simulink model "Lombardini_dual_fuel"  (R2024b)
settings: Solver=FixedStepAuto  StartTime=0.0  StopTime=2000  RelTol=1e-3  EnableMultiTasking=on
PreLoadFcn:
  | try, eval([bdroot '_setup']); catch, eval('model_setup', ''); end
InitFcn:
  | try, eval([bdroot '_setup']); catch, eval('model_setup', ''); end
model workspace (MAT data in the model file):
  PID_rpm = [1000 2000 3000 4000]
undefined symbols (not defined in the file): ECU555, motohawk_build_version, motohawk_get_target_image, motohawk_target_type, motohawk_trunc_name, motohawk_vardec_path
libraries: MotoHawk_lib x118, motohawk_annotations_lib x23, dspstat3 x13, motohawk_examples_lib x1, MotoHawk_Protocols_lib x1
(part 1 of 5)
CloseFcn:
  | try, eval([bdroot '_close']); catch, eval('model_close', ''); end
Description:
  | Lombardini_dual_fuel
settings Model: MotoHawkBuildVersion=000  MotoHawkBuildStats=struct('TotalFLASH',{0},'TotalEEPROM',{0},'TotalRAM',{0},'AppFLASH',{0},'AppEEPROM',{0},'AppRAM',{0},'HeapRAM',{0},'BuildSuccessCount',{0},'BuildErrorCount',{0})  MotoHawkModelSavedName=Lombardini_dual_fuel  MotoHawkModelGUID=DD803FFC-3B74-4B09-85B7-E854500213FD  MotoHawkModelOpenTime=2025 8 5 14 36 14.209  MotoHawkModelElapsedTime=1228077.779  MotoHawkBuildInfo=struct('model_name',{'motohawk_template_model'},'motohawk_version',{'0.8.4_beta1'},'motohawk_component_version',{'0.0.3'},'matlab_version',{'6.5.1'},'build_version',{'000'},'layout_type',{'DEV'},'eri_table0_rev',{9},'max_eri_table_size',{255},'fptype',{0},'fgnd_base_period_ms',{5},'bgnd_base_period_ms',{50},'module_type',{'ECU555-80'},'processor_family',{'PPC'},'processor_type',{'MPC555'},'toolchain',{'GHS3.6'},'component',{0},'resource_file',{'PCM555Resources.h'},'archive_file',{'PCM.a'},'enable_build',{1},'flash_size',{458752},'ee_size',{8192},'ram_size',{26624},'decram_size',{0},'module_memory_def',{'MPC555_ModMemoryDef_Dev'},'use_debug_vardecs',{1},'root_build_dir',{'C:\MotoTron\MOTOHA~3\Blocks\Project'},'build_dir',{'C:\MotoTron\MOTOHA~3\Blocks\Project\motohawk_template_model_Build'},'dll_name',{'motohawk__000'},'srz_name',{'motohawk_template_model_000'},'fgnd_stack_size',{3072},'fgnd_angle_stack_size',{0},'bgnd_stack_size',{2048},'idle_stack_size',{1024},'irq_stack_size',{1536},'heap_size',{4096},'install_dll_dir',{'C:\ECUFiles\TDBDLL\'},'install_srz_dir',{'C:\ECUFiles\Programs\'},'motodevelopment_dir',{'C:\PROGRA~1\MotoTron\DEVELO~1\'},'motohawk_dir',{'C:\MotoTron\MOTOHA~3'},'ghs_dir',{'C:\GHS\ppc36'},'cw_dir',{'C:\Program Files\Freescale\CW for HC12 V4.5'},'matlab_root',{'C:\MATLAB6p5p1'},'model_guid',{'a528c725-4135-4734-9f-2c-07-29-37-5b-38'},'build_guid',{[]},'token_guid',{'6198A7A8FF044D4685C525ADFA06DAD5'})  MotoHawkBuildDirectory=C:\Users\ASUS\MATLAB\Projects\Lombardini_Hybrid\models\Lombardini_dual_fuel_Build  MotoHawkTargetDefnBlock=Lombardini_dual_fuel/motohawk_target_def1  MotoHawkCANInfo=struct('DefnArr',{struct('res_name',{'CAN_1'},'text_resource',{'(None)'},'IsSupportedMethodArr',{logical([0;0;0;0;0;0;0;0;0;0;0;0;0;0;0;0;0])})})  Creator=cspenc  LastModifiedBy=ASUS
settings ConfigSet: Description="This Simulink Configuration Set is preconfigured  for the MotoHawk target \"ECU555-48-0403\"."
settings SolverCC: AlgebraicLoopSolver=TrustRegion  AutoInsertRateTranBlk=on
settings DataIOCC: LimitDataPoints=on  SaveFormat=Array  ReturnWorkspaceOutputs=off
settings OptimizationCC: DefaultParameterBehavior=Inlined  InlineInvariantSignals=on  EnhancedBackFolding=on  InitFltsAndDblsToZero=on  NoFixptDivByZeroProtection=on  EfficientFloat2IntCast=on  LifeSpan=1  EfficientTunableParamExpr=on
settings DebuggingCC: AlgebraicLoopMsg=none  MergeDetectMultiDrivingBlocksExec=none  InheritedTsInSrcMsg=none  TasksWithSamePriorityMsg=none  ParamSuppressDoubleToSinglePrecisionLossMsg=on  ParamPrecisionLossAbsoluteDiffThreshold=0.5  UnconnectedInputMsg=warning  UnconnectedOutputMsg=warning  UnconnectedLineMsg=warning  ModelReferenceIOMismatchMessage=warning  SFUnexpectedBacktrackingDiag=warning  SFNoUnconditionalDefaultTransitionDiag=warning  SFExecutionAtInitializationDiag=none  UnitsInconsistencyMsg=none  ArithmeticOperatorsInVariantConditions=warning
settings HardwareCC: ProdBitPerPointer=32  ProdBitPerSizeT=32  ProdBitPerPtrDiffT=32  ProdLargestAtomicInteger=Integer  ProdIntDivRoundTo=Undefined  ProdEndianess=BigEndian  ProdWordSize=32  ProdHWDeviceType=Specified
settings ModelReferenceCC: UpdateModelReferenceTargets=IfOutOfDate  EnableRefExpFcnMdlSchedulingChecks=on  CheckModelReferenceTargetMessage=warning  ModelReferenceNumInstancesAllowed=Single  PropagateSignalLabelsOutOfModel=off
settings SFSimCC: SimCustomHeaderCode="#include \"FuelControl.h\""  SimUserSources=Code/Fuelcontrol.c  SimUserIncludeDirs=Code  SimUseLocalCustomCode=off  MATLABDynamicMemAlloc=off  CustomCodeUndefinedFunction=UseInterfaceOnly
settings RTWCC: Description=MotoHawk(tm) Rapid Prototyping  SystemTargetFile=motohawk_ert_rtw.tlc  MakeCommand=make_rtw_motohawk  TemplateMakefile=motohawk_ert_rtw.tmf  RTWUseLocalCustomCode=off  GPUComputeCapability=3.5
settings CodeAppCC: IgnoreCustomStorageClasses=off  MaxIdLength=100  CustomSymbolStrType=$N$R$M  CustomSymbolStrField=$H$N$M  StateflowObjectComments=on  InternalIdentifier=Classic
settings STFCustomTargetCC: MultiwordTypeDef=User defined  MultiwordLength=0  IncludeMdlTerminateFcn=off  CombineOutputUpdateFcns=on  SuppressErrorStatus=on  ERTCustomFileBanners=on  SupportContinuousTime=off  SupportNonInlinedSFcns=off  RemoveResetFunc=on  MATLABClassNameForMDSCustomization=Simulink.SoftwareTarget.ERTCustomization  SystemTargetFile=motohawk_ert_rtw.tlc
settings ERTTargetCC: MultiwordTypeDef=User defined  MultiwordLength=0  ParMdlRefBuildCompliant=off  CompOptLevelCompliant=off  ConcurrentExecutionCompliant=off  IncludeMdlTerminateFcn=off  SuppressErrorStatus=on  ModelStepFunctionPrototypeControlCompliant=off  CPPClassGenCompliant=off  UseToolchainInfoCompliant=off  ERTCustomFileTemplate=motohawk_file_process.tlc  ConvertIfToSwitch=off  SuppressUnreachableDefaultCases=off  DynamicArrayContainerType=coder::array
settings ConfigComp: CovMetricSettings=dw  CovSaveCumulativeToWorkspaceVar=on  CovSaveSingleToWorkspaceVar=on  CovExternalEMLEnable=off  CovSFcnEnable=off

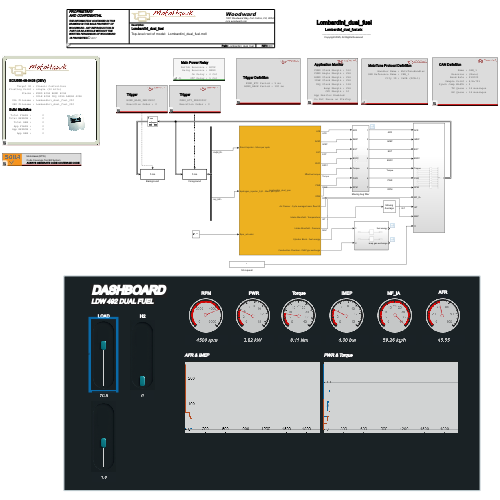
[thumbnail: Simulink's stored preview of the top-level diagram]
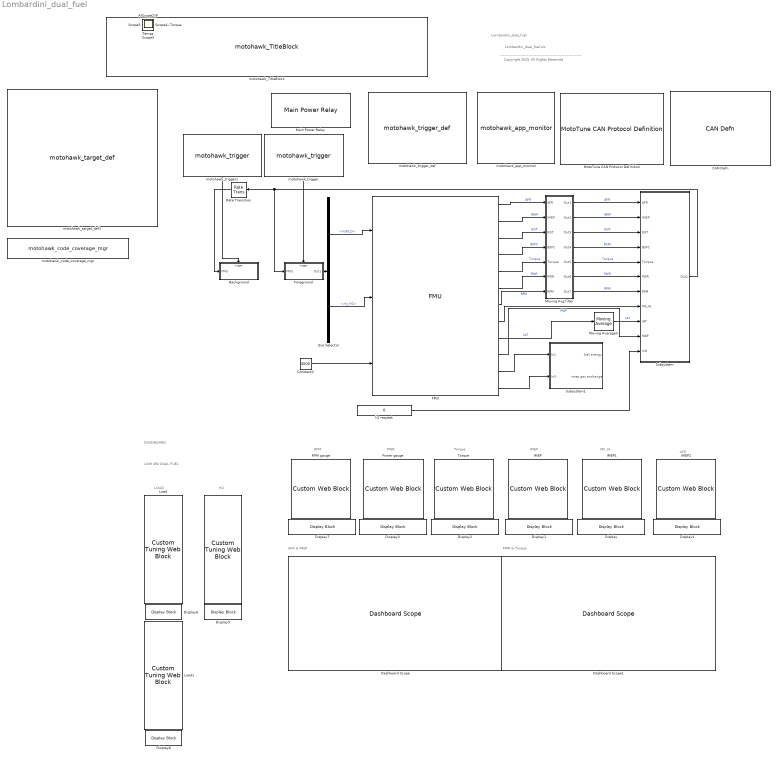
== system Lombardini_dual_fuel ==
  note: RPM
  note: Lombardini_dual_fuel
  note: Lombardini_dual_fuel.slx
  note: -------------------------------------------------------------
  note: Copyright 2025, All Rights Reserved
  note: PWR
  note: Torque
  note: IMEP
  note: MF_IA
  note: AFR
  note: LOAD
  note: H2
  note: DASHBOARD
  note: AFR & IMEP
  note: PWR & Torque
  note: LDW 492 DUAL FUEL
  . : CustomTuningWebBlock  LabelPosition=Hide  ShowInitialText=on  Configuration="{\"components\":[{\"name\":\"LinearScaleComponent\",\"settings\":{\"bounds\":{\"max\":1,\"min\":0,\"tickInterval\":\"auto\"},\"internalTickHeightScaleFactor\":0.66,\"labelColor\":[255,255,255],\"labelFont\":{\"font\":\"Arial\",\"fontSize\":12},\"labelOffset\":0.054,\"labelTransparency\":1,\"needleImage\":{\"size\":[216,346],\"src\":\"data:image\\/jpeg;base64,\\/9j\\/60nfSlCyAAAAAAEAAEnVanVtYgAAAB5qdW1kYzJwYQARABCAAACqADibcQNjMnBhAAAANxNqdW1iAAAAR2p1bWRjMm1hABEAEIAAAKoAOJtxA3VybjpjMnBhOmZjZjA1MzM0LWQyMmQtNGI4ZS1iN2VjLWNjYWE3OTFmMGZhNgAAAAHhanVtYgAAAClqdW1kYzJhcwARABCAAACqADibcQNjMnBhLmFzc2VydGlvbnMAAAABBWp1bWIAAAApanVtZGNib3IAEQAQgAAAqgA4m3EDYzJwYS5hY3Rpb25zLnYyAAAAANRjYm9yoWdhY3Rpb25zgqNmYWN0aW9ubGMycGEuY3JlYXRlZG1zb2Z0d2FyZUFnZW50v2RuYW1lZkdQVC00b\\/ ...(+43706 chars)\",\"srcOrientation\":\"Down\"},\"needleOffset\":[-0.2905073649754501,-0.22009935040122278],\"needleSize\":{\"height\":0.15292477116704806,\"width\":0.26725898692810457},\"position\":[0.07772988505747126,0.2764501633986928,0.6154003267973857,0.8782327586206896],\"referencePoint\":\"auto\",\"scaleColors\":[],\"scaleColorsSize\":0.2,\"scaleDirection\":\"BT\",\"showLabels\":false,\"showMinorTicks\":0,\"showSpanLine\":false,\"showTicks\":false,\"tickColor\":[26,33,36],\"tickTransparency\":1,\"valueBarColor\":[255,255,255],\"valueBarOffset\":0.12,\"valueBarSize\":0.1,\"valueBarTransparency\":1}},{\"name\":\"BackgroundImageComponent\",\"settings\":{\"image\":{\"size\":[512,1450],\"src\":\"data:image\\/jpeg;base64,\\/9j\\/60GWSlCJAAAAAAEAAEGManVtYgAAAB5qdW1kYzJwYQARABCAAACqADibcQNjMnBhAAAANxNqdW1iAAAAR2p1bWRjMm1hABEAEIAAAKoAOJtxA3VybjpjMnBhOmZjZjA1MzM0LWQyMmQtNGI4ZS1iN2VjLWNjYWE3OTFmMGZhNgAAAAHhanVtYgAAAClqdW1kYzJhcwARABCAAACqADibcQNjMnBhLmFzc2VydGlvbnMAAAABBWp1bWIAAAApanVtZGNib3IAEQAQgAAAqgA4m3EDYzJwYS5hY3Rpb25zLnYyAAAAANRjYm9yoWdhY3Rpb25zgqNmYWN0aW9ubGMycGEuY3JlYXRlZG1zb2Z0d2FyZUFnZW50v2RuYW1lZkdQVC00b\\/ ...(+77138 chars)\",\"srcOrientation\":\"Down\"},\"position\":[0,0,1,1],\"scaleMode\":\"0\"}},{\"name\":\"ForegroundImageComponent\",\"settings\":{\"image\":{\"size\":[0,0],\"src\":\"default\",\"srcOrientation\":\"Down\"},\"isForeground\":1,\"position\":[0,0,1,1],\"scaleMode\":\"0\"}}],\"settings\":{\"BindingType\":\"param\",\"aspectRatio\":3.7777777777777777,\"backgroundColor\":[0,0,0,\"1\"],\"backgroundOffset\":0.4,\"backgroundOpacity\":1,\"fixedAspectRatio\":\"on\",\"foregroundColor\":[252,252,196],\"orientation\":\"vertical\",\"showBackgroundColor\":false,\"value\":0,\"version\":\"R2023a\"},\"type\":\"LinearGauge\"}"  CustomBackgroundColor="{\"color\":[0.0196078431372549,0.5450980392156862,0.5490196078431373],\"show\":false}"
  Background : Subsystem  TreatAsAtomicUnit=on
      mask init:
      | SampleTime = 0.005;
      | lbl = sprintf('%d ms', SampleTime * 1000);
      settings: RTWSystemCode=Nonreusable function  RTWFcnNameOpts=Use subsystem name  RTWFileNameOpts=Use function name
      mask Display: disp(lbl);
  Bus Selector : BusSelector  OutputSignals=InjM_D,inj_H2
  CAN Defn : MotoHawk_lib/CAN Blocks/CAN Defn  Priority=-100  res_name='CAN_1'  text_resource=(None)  target=ECU555-48-0403  bit_time_src=Default  update_without_reboot=off  btime=250000  baud_rate_src=Constant (Edit Field)  baud_rate=uint32(250000)  baud_rate_data_store_name='CAN1_BaudRate'  sample_point_tq_src=Constant (Popup)  sample_point_tq=6  sample_point_tq_edit=6  sample_point_tq_data_store_name='SamplePoint_TQ'  total_tq_src=Constant (Popup)  total_tq=8  total_tq_edit=8  total_tq_data_store_name='Total_TQ'  synch_jw_src=Constant (Popup)  synch_jw=1  synch_jw_edit=2  synch_jw_data_store_name='SynchJumpWidth'  tx_queue_size=16  rx_queue_size=16  recieve_transmitted_messages=on  use_rx_dispatch_task=off  rx_dispatch_task_name='ApplicationInterruptTask'  use_frameratelimit=off  frameratelimit_src=Constant  frameratelimit_value=5000  frameratelimit_data_store_name='FrameRateLimit'  use_can_fd=off  max_fd_frame_size=8  use_fast_bit_timing=off  fast_bit_time_src=Default  fast_btime=500000  fast_bit_rate_src=Constant (Edit Field)  fast_bit_rate=1000000  fast_bit_rate_data_store_name='FastBit_DataStoreName'  fast_bit_sample_point_tq_src=Constant (Edit Field)  fast_bit_sample_point_tq=6  fast_bit_sample_point_tq_data_store_name='FastBitTQ_DataStoreName'  fast_bit_total_tq_src=Constant (Edit Field)  fast_bit_total_tq=8  fast_bit_total_tq_data_store_name='FastBitTotal_TQ_DataStoreName'  fast_bit_sync_jump_width_src=Constant (Edit Field)  fast_bit_sync_jump_width=2  fast_bit_sync_jump_width_data_store_name='FastBitSyncJumpWidth_DataStoreName'
      settings: SourceProductName=MotoHawk
  Constant2 : Constant  Value=4500
  Dashboard Scope : DashboardScope  Ymin=0  Ymax=60  LegendPosition=Hide  TicksPosition=Inside
      settings: Grid=Horizontal
  Dashboard Scope1 : DashboardScope  Ymin=0  Ymax=30  LegendPosition=Hide  TicksPosition=Inside
      settings: Grid=Horizontal
  Display : DisplayBlock  LabelPosition=Hide  Format=Custom  Transparency=1  FormatString=%.2f kg/h
  Display1 : DisplayBlock  LabelPosition=Hide  Format=Custom  Transparency=1  FormatString=%.2f bar
  Display2 : DisplayBlock  LabelPosition=Hide  Format=Custom  Transparency=1  FormatString=%.2f Nm
  Display3 : DisplayBlock  LabelPosition=Hide  Format=Custom  Transparency=1  FormatString=%.2f kW
  Display4 : DisplayBlock  LabelPosition=Hide  Format=Custom  Transparency=1  FormatString=%.2f
  Display5 : DisplayBlock  LabelPosition=Hide  Format=Custom  Transparency=1  FormatString=%i
  Display6 : DisplayBlock  LabelPosition=Hide  Format=Custom  Transparency=1  FormatString=%.1f
  Display7 : DisplayBlock  LabelPosition=Hide  Format=Custom  Transparency=1  FormatString=%.0f rpm
  Display8 : DisplayBlock  LabelPosition=Hide  Format=Custom  Transparency=1  FormatString=%.1f
  FMU : FMU  FMUName=Lombardini_dual_rpm.fmu  FMUDebugLogging=on  FMUDebugLoggingRedirect=Display  FMUMode=CoSimulation  FMUInitializeEnumObject=off  FMUCachedDialogLayout="{\"Geometry\":[1021,8,891,1016],\"ParameterColumnsWidthConfig\":\"{\\\"columns\\\":[{\\\"name\\\":\\\"Parameter\\\",\\\"width\\\":73},{\\\"name\\\":\\\"Value\\\",\\\"width\\\":44},{\\\"name\\\":\\\"Unit\\\",\\\"width\\\":36},{\\\"name\\\":\\\"Description\\\",\\\"width\\\":79}]}\",\"InputColumnsWidthConfig\":\"{\\\"columns\\\":[{\\\"name\\\":\\\"Name\\\",\\\"width\\\":198},{\\\"name\\\":\\\"Visibility\\\",\\\"width\\\":49},{\\\"name\\\":\\\"Start\\\",\\\"width\\\":190},{\\\"name\\\":\\\"Unit\\\",\\\"width\\\":186},{\\\"name\\\":\\\"Type Object\\\",\\\"width\\\":233}]}\",\"OutputColumnsWidthConfig\":\"{\\\"columns\\\":[{\\\"name\\\":\\\"Name\\\",\\\"width\\\":48},{\\\"name\\\":\\\"Visibility\\\",\\\"width\\\":60},{\\\"name\\\":\\\"Start\\\",\\\"width\\\":40},{\\\"name\\\":\\\"Unit\\\",\\\"width\\\":36},{\\\"name\\\":\\\"Type Object\\\",\\\"width\\\":82}]}\"}"  Solver_Disable_outputs=off  mask(Lombardini_dual_rpm [Co-Simulation, v2.0]){}
      mask Display:
      | disp('Lombardini_dual_rpm');
      | port_label('output',1,'AFR');
      | port_label('output',2,'IMEP');
      | port_label('output',3,'EGT');
      | port_label('output',4,'BSFC');
      | port_label('output',5,'Effective torque');
      | port_label('output',6,'PWR');
      | port_label('output',7,'RPM');
      | port_label('output',8,'Air Cleaner - Cycle averaged mass flow US');
      | port_label('output',9,'Intake Manifold - Temperature');
      | port_label('output',10,'Intake Manifold - Pressure');
      | port_label('output',11,'Cylinder Block - Fuel energy');
      | port_label('output',12,'Combustion Chamber - IMEP gas exchange');
      | port_label('input',1,'Direct Injector - Mass per cycle');
      | port_label('input',2,'Hydrogen_injector_Cyl1 - Mass per cycle');
      | port_label('input',3,'Rpm_actuator');
  Foreground : Subsystem  TreatAsAtomicUnit=on
      mask init:
      | SampleTime = 0.005;
      | lbl = sprintf('%d ms', SampleTime * 1000);
      settings: RTWSystemCode=Nonreusable function  RTWFcnNameOpts=Use subsystem name  RTWFileNameOpts=Use function name
      mask Display: disp(lbl);
  IMEP : CustomWebBlock  LabelPosition=Hide  ShowInitialText=on  Configuration="{\"components\":[{\"name\":\"CircularScaleComponent\",\"settings\":{\"bounds\":{\"max\":15,\"min\":0,\"tickInterval\":\"auto\"},\"direction\":\"cw\",\"flipLimits\":0,\"innerRadius\":0.75,\"internalTickHeightScaleFactor\":1,\"labelColor\":[128,128,128],\"labelFont\":{\"font\":\"Arial\",\"fontSize\":12},\"labelRadius\":0.528,\"labelTransparency\":1,\"minorTickHeightScaleFactor\":0.2,\"needleImage\":{\"size\":[200,50],\"src\":\"data:image\\/svg+xml;base64,PD94bWwgdmVyc2lvbj0iMS4wIiBlbmNvZGluZz0idXRmLTgiPz4KPCEtLSBHZW5lcmF0b3I6IEFkb2JlIElsbHVzdHJhdG9yIDI0LjEuMiwgU1ZHIEV4cG9ydCBQbHVnLUluIC4gU1ZHIFZlcnNpb246IDYuMDAgQnVpbGQgMCkgIC0tPgo8c3ZnIHZlcnNpb249IjEuMSIgaWQ9IkxheWVyXzEiIHhtbG5zPSJodHRwOi8vd3d3LnczLm9yZy8yMDAwL3N2ZyIgeG1sbnM6eGxpbms9Imh0dHA6Ly93d3cudzMub3JnLzE5OTkveGxpbmsiIHg9IjBweCIgeT0iMHB4IgoJIHZpZXdCb3g9IjAgMCAyMDAgNTAiIHN0eWxlPSJlbmFibGUtYmFja2dyb3VuZDpuZXcgMCAwIDIwMCA1MDsiIHhtbDpzcGFjZT0icHJlc2VydmUiPgo8c3R5bGUgdHlwZT0idGV4dC9jc3MiPgoJLnN0MHtmaWxsOiNFQzIxMjc7fQo8L3N0eWxlPgo8cGF0aCBjbGFzcz0ic3QwIiBkPSJNMTYyLjgsMTMuN0MxNjksNC40LDE4MS43LDEuOSwxOTEsOC4xczExLjgsMTguOSw1LjYsMjguMnMtMTguOSwxMS44LTI4LjIsNS42bDAsMAoJQzE1OS4xLDM1LjYsMTU2LjYsMjMsMTYyLjgsMTMuN0wxNjIuOCwxMy43eiBNMTY1LjgsMTUuOGMtNS4xLDcuNi0zLjEsMTcuOSw0LjYsMjNjNy42LDUuMSwxNy45LDMuMSwyMy00LjYKCWM1LjEtNy42LDMuMS0xNy45LTQuNi0yM2wwLDBDMTgxLjIsNi4yLDE3MC45LDguMiwxNjUuOCwxNS44eiIvPgo8cGF0aCBjbGFzcz0ic3QwIiBkPSJNMC40LDI1Ljl2LTMuM2wxNTktMi41Yy0wLjcsMi42LTAuNyw1LjIsMCw3LjhMMC40LDI1Ljl6Ii8+CjxjaXJjbGUgY2xhc3M9InN0MCIgY3g9IjE3OS42IiBjeT0iMjQiIHI9IjAuNyIvPgo8L3N2Zz4K\"},\"needleOffset\":[0.18464878250906522,0],\"needleOrientation\":-45,\"needleRotation\":180,\"needleSize\":{\"height\":0.11741692305346914,\"width\":0.46108337545091255},\"outerRadius\":0.9,\"position\":[0.05,0.05,0.9,0.9],\"referencePoint\":\"auto\",\"scaleAngle\":270,\"scaleAngleOffset\":135,\"scaleColors\":[],\"scaleColorsSize\":0.2,\"scaleDirection\":\"CW\",\"scalePosition\":[0,0,1,1],\"showLabels\":1,\"showMinorTicks\":1,\"showSpanLine\":1,\"showTicks\":1,\"tickColor\":[38,38,38],\"tickTransparency\":1,\"valueBarColor\":[255,0,0],\"valueBarPosition\":[0,0,1,1],\"valueBarSize\":0.2,\"valueBarTransparency\":1}},{\"name\":\"BackgroundImageComponent\",\"settings\":{\"image\":{\"size\":[500,500],\"src\":\"data:image\\/svg+xml;base64,PD94bWwgdmVyc2lvbj0iMS4wIiBlbmNvZGluZz0iVVRGLTgiIHN0YW5kYWxvbmU9Im5vIj8+CjxzdmcKICAgeG1sbnM6ZGM9Imh0dHA6Ly9wdXJsLm9yZy9kYy9lbGVtZW50cy8xLjEvIgogICB4bWxuczpjYz0iaHR0cDovL2NyZWF0aXZlY29tbW9ucy5vcmcvbnMjIgogICB4bWxuczpyZGY9Imh0dHA6Ly93d3cudzMub3JnLzE5OTkvMDIvMjItcmRmLXN5bnRheC1ucyMiCiAgIHhtbG5zOnN2Zz0iaHR0cDovL3d3dy53My5vcmcvMjAwMC9zdmciCiAgIHhtbG5zPSJodHRwOi8vd3d3LnczLm9yZy8yMDAwL3N2ZyIKICAgeG1sbnM6 ...(+9964 chars)\"},\"position\":[0,0,1,1],\"scaleMode\":\"0\"}},{\"name\":\"ForegroundImageComponent\",\"settings\":{\"image\":{\"size\":[0,0],\"src\":\"default\",\"srcOrientation\":[]},\"isForeground\":1,\"position\":[0,0,1,1],\"scaleMode\":\"0\"}}],\"settings\":{\"BindingType\":\"signal\",\"aspectRatio\":1.032258064516129,\"backgroundColor\":[0,0,0,\"1\"],\"backgroundOffset\":1,\"backgroundOpacity\":1,\"direction\":\"cw\",\"fixedAspectRatio\":\"on\",\"flipLimits\":0,\"orientation\":\"horizontal\",\"showBackgroundColor\":false,\"value\":0,\"version\":\"R2023a\"},\"type\":\"CircularGauge\"}"  CustomBackgroundColor="{\"color\":[0.9411764705882353,0.9411764705882353,0.9411764705882353],\"show\":true}"
  IMEP1 : CustomWebBlock  LabelPosition=Hide  ShowInitialText=on  Configuration="{\"components\":[{\"name\":\"CircularScaleComponent\",\"settings\":{\"bounds\":{\"max\":40,\"min\":0,\"tickInterval\":\"auto\"},\"direction\":\"cw\",\"flipLimits\":0,\"innerRadius\":0.75,\"internalTickHeightScaleFactor\":1,\"labelColor\":[128,128,128],\"labelFont\":{\"font\":\"Arial\",\"fontSize\":12},\"labelRadius\":0.528,\"labelTransparency\":1,\"minorTickHeightScaleFactor\":0.2,\"needleImage\":{\"size\":[200,50],\"src\":\"data:image\\/svg+xml;base64,PD94bWwgdmVyc2lvbj0iMS4wIiBlbmNvZGluZz0idXRmLTgiPz4KPCEtLSBHZW5lcmF0b3I6IEFkb2JlIElsbHVzdHJhdG9yIDI0LjEuMiwgU1ZHIEV4cG9ydCBQbHVnLUluIC4gU1ZHIFZlcnNpb246IDYuMDAgQnVpbGQgMCkgIC0tPgo8c3ZnIHZlcnNpb249IjEuMSIgaWQ9IkxheWVyXzEiIHhtbG5zPSJodHRwOi8vd3d3LnczLm9yZy8yMDAwL3N2ZyIgeG1sbnM6eGxpbms9Imh0dHA6Ly93d3cudzMub3JnLzE5OTkveGxpbmsiIHg9IjBweCIgeT0iMHB4IgoJIHZpZXdCb3g9IjAgMCAyMDAgNTAiIHN0eWxlPSJlbmFibGUtYmFja2dyb3VuZDpuZXcgMCAwIDIwMCA1MDsiIHhtbDpzcGFjZT0icHJlc2VydmUiPgo8c3R5bGUgdHlwZT0idGV4dC9jc3MiPgoJLnN0MHtmaWxsOiNFQzIxMjc7fQo8L3N0eWxlPgo8cGF0aCBjbGFzcz0ic3QwIiBkPSJNMTYyLjgsMTMuN0MxNjksNC40LDE4MS43LDEuOSwxOTEsOC4xczExLjgsMTguOSw1LjYsMjguMnMtMTguOSwxMS44LTI4LjIsNS42bDAsMAoJQzE1OS4xLDM1LjYsMTU2LjYsMjMsMTYyLjgsMTMuN0wxNjIuOCwxMy43eiBNMTY1LjgsMTUuOGMtNS4xLDcuNi0zLjEsMTcuOSw0LjYsMjNjNy42LDUuMSwxNy45LDMuMSwyMy00LjYKCWM1LjEtNy42LDMuMS0xNy45LTQuNi0yM2wwLDBDMTgxLjIsNi4yLDE3MC45LDguMiwxNjUuOCwxNS44eiIvPgo8cGF0aCBjbGFzcz0ic3QwIiBkPSJNMC40LDI1Ljl2LTMuM2wxNTktMi41Yy0wLjcsMi42LTAuNyw1LjIsMCw3LjhMMC40LDI1Ljl6Ii8+CjxjaXJjbGUgY2xhc3M9InN0MCIgY3g9IjE3OS42IiBjeT0iMjQiIHI9IjAuNyIvPgo8L3N2Zz4K\"},\"needleOffset\":[0.18464878250906522,0],\"needleOrientation\":-45,\"needleRotation\":180,\"needleSize\":{\"height\":0.11741692305346914,\"width\":0.46108337545091255},\"outerRadius\":0.9,\"position\":[0.05,0.05,0.9,0.9],\"referencePoint\":\"auto\",\"scaleAngle\":270,\"scaleAngleOffset\":135,\"scaleColors\":[],\"scaleColorsSize\":0.2,\"scaleDirection\":\"CW\",\"scalePosition\":[0,0,1,1],\"showLabels\":1,\"showMinorTicks\":1,\"showSpanLine\":1,\"showTicks\":1,\"tickColor\":[38,38,38],\"tickTransparency\":1,\"valueBarColor\":[255,0,0],\"valueBarPosition\":[0,0,1,1],\"valueBarSize\":0.2,\"valueBarTransparency\":1}},{\"name\":\"BackgroundImageComponent\",\"settings\":{\"image\":{\"size\":[500,500],\"src\":\"data:image\\/svg+xml;base64,PD94bWwgdmVyc2lvbj0iMS4wIiBlbmNvZGluZz0iVVRGLTgiIHN0YW5kYWxvbmU9Im5vIj8+CjxzdmcKICAgeG1sbnM6ZGM9Imh0dHA6Ly9wdXJsLm9yZy9kYy9lbGVtZW50cy8xLjEvIgogICB4bWxuczpjYz0iaHR0cDovL2NyZWF0aXZlY29tbW9ucy5vcmcvbnMjIgogICB4bWxuczpyZGY9Imh0dHA6Ly93d3cudzMub3JnLzE5OTkvMDIvMjItcmRmLXN5bnRheC1ucyMiCiAgIHhtbG5zOnN2Zz0iaHR0cDovL3d3dy53My5vcmcvMjAwMC9zdmciCiAgIHhtbG5zPSJodHRwOi8vd3d3LnczLm9yZy8yMDAwL3N2ZyIKICAgeG1sbnM6 ...(+9964 chars)\"},\"position\":[0,0,1,1],\"scaleMode\":\"0\"}},{\"name\":\"ForegroundImageComponent\",\"settings\":{\"image\":{\"size\":[0,0],\"src\":\"default\",\"srcOrientation\":[]},\"isForeground\":1,\"position\":[0,0,1,1],\"scaleMode\":\"0\"}}],\"settings\":{\"BindingType\":\"signal\",\"aspectRatio\":1.032258064516129,\"backgroundColor\":[0,0,0,\"1\"],\"backgroundOffset\":1,\"backgroundOpacity\":1,\"direction\":\"cw\",\"fixedAspectRatio\":\"on\",\"flipLimits\":0,\"orientation\":\"horizontal\",\"showBackgroundColor\":false,\"value\":0,\"version\":\"R2023a\"},\"type\":\"CircularGauge\"}"  CustomBackgroundColor="{\"color\":[0.9411764705882353,0.9411764705882353,0.9411764705882353],\"show\":true}"
  IMEP2 : CustomWebBlock  LabelPosition=Hide  ShowInitialText=on  Configuration="{\"components\":[{\"name\":\"CircularScaleComponent\",\"settings\":{\"bounds\":{\"max\":100,\"min\":0,\"tickInterval\":\"auto\"},\"direction\":\"cw\",\"flipLimits\":0,\"innerRadius\":0.75,\"internalTickHeightScaleFactor\":1,\"labelColor\":[128,128,128],\"labelFont\":{\"font\":\"Arial\",\"fontSize\":12},\"labelRadius\":0.528,\"labelTransparency\":1,\"minorTickHeightScaleFactor\":0.2,\"needleImage\":{\"size\":[200,50],\"src\":\"data:image\\/svg+xml;base64,PD94bWwgdmVyc2lvbj0iMS4wIiBlbmNvZGluZz0idXRmLTgiPz4KPCEtLSBHZW5lcmF0b3I6IEFkb2JlIElsbHVzdHJhdG9yIDI0LjEuMiwgU1ZHIEV4cG9ydCBQbHVnLUluIC4gU1ZHIFZlcnNpb246IDYuMDAgQnVpbGQgMCkgIC0tPgo8c3ZnIHZlcnNpb249IjEuMSIgaWQ9IkxheWVyXzEiIHhtbG5zPSJodHRwOi8vd3d3LnczLm9yZy8yMDAwL3N2ZyIgeG1sbnM6eGxpbms9Imh0dHA6Ly93d3cudzMub3JnLzE5OTkveGxpbmsiIHg9IjBweCIgeT0iMHB4IgoJIHZpZXdCb3g9IjAgMCAyMDAgNTAiIHN0eWxlPSJlbmFibGUtYmFja2dyb3VuZDpuZXcgMCAwIDIwMCA1MDsiIHhtbDpzcGFjZT0icHJlc2VydmUiPgo8c3R5bGUgdHlwZT0idGV4dC9jc3MiPgoJLnN0MHtmaWxsOiNFQzIxMjc7fQo8L3N0eWxlPgo8cGF0aCBjbGFzcz0ic3QwIiBkPSJNMTYyLjgsMTMuN0MxNjksNC40LDE4MS43LDEuOSwxOTEsOC4xczExLjgsMTguOSw1LjYsMjguMnMtMTguOSwxMS44LTI4LjIsNS42bDAsMAoJQzE1OS4xLDM1LjYsMTU2LjYsMjMsMTYyLjgsMTMuN0wxNjIuOCwxMy43eiBNMTY1LjgsMTUuOGMtNS4xLDcuNi0zLjEsMTcuOSw0LjYsMjNjNy42LDUuMSwxNy45LDMuMSwyMy00LjYKCWM1LjEtNy42LDMuMS0xNy45LTQuNi0yM2wwLDBDMTgxLjIsNi4yLDE3MC45LDguMiwxNjUuOCwxNS44eiIvPgo8cGF0aCBjbGFzcz0ic3QwIiBkPSJNMC40LDI1Ljl2LTMuM2wxNTktMi41Yy0wLjcsMi42LTAuNyw1LjIsMCw3LjhMMC40LDI1Ljl6Ii8+CjxjaXJjbGUgY2xhc3M9InN0MCIgY3g9IjE3OS42IiBjeT0iMjQiIHI9IjAuNyIvPgo8L3N2Zz4K\"},\"needleOffset\":[0.18464878250906522,0],\"needleOrientation\":-45,\"needleRotation\":180,\"needleSize\":{\"height\":0.11741692305346914,\"width\":0.46108337545091255},\"outerRadius\":0.9,\"position\":[0.05,0.05,0.9,0.9],\"referencePoint\":\"auto\",\"scaleAngle\":270,\"scaleAngleOffset\":135,\"scaleColors\":[],\"scaleColorsSize\":0.2,\"scaleDirection\":\"CW\",\"scalePosition\":[0,0,1,1],\"showLabels\":1,\"showMinorTicks\":1,\"showSpanLine\":1,\"showTicks\":1,\"tickColor\":[38,38,38],\"tickTransparency\":1,\"valueBarColor\":[255,0,0],\"valueBarPosition\":[0,0,1,1],\"valueBarSize\":0.2,\"valueBarTransparency\":1}},{\"name\":\"BackgroundImageComponent\",\"settings\":{\"image\":{\"size\":[500,500],\"src\":\"data:image\\/svg+xml;base64,PD94bWwgdmVyc2lvbj0iMS4wIiBlbmNvZGluZz0iVVRGLTgiIHN0YW5kYWxvbmU9Im5vIj8+CjxzdmcKICAgeG1sbnM6ZGM9Imh0dHA6Ly9wdXJsLm9yZy9kYy9lbGVtZW50cy8xLjEvIgogICB4bWxuczpjYz0iaHR0cDovL2NyZWF0aXZlY29tbW9ucy5vcmcvbnMjIgogICB4bWxuczpyZGY9Imh0dHA6Ly93d3cudzMub3JnLzE5OTkvMDIvMjItcmRmLXN5bnRheC1ucyMiCiAgIHhtbG5zOnN2Zz0iaHR0cDovL3d3dy53My5vcmcvMjAwMC9zdmciCiAgIHhtbG5zPSJodHRwOi8vd3d3LnczLm9yZy8yMDAwL3N2ZyIKICAgeG1sbnM6 ...(+9964 chars)\"},\"position\":[0,0,1,1],\"scaleMode\":\"0\"}},{\"name\":\"ForegroundImageComponent\",\"settings\":{\"image\":{\"size\":[0,0],\"src\":\"default\",\"srcOrientation\":[]},\"isForeground\":1,\"position\":[0,0,1,1],\"scaleMode\":\"0\"}}],\"settings\":{\"BindingType\":\"signal\",\"aspectRatio\":1.032258064516129,\"backgroundColor\":[0,0,0,\"1\"],\"backgroundOffset\":1,\"backgroundOpacity\":1,\"direction\":\"cw\",\"fixedAspectRatio\":\"on\",\"flipLimits\":0,\"orientation\":\"horizontal\",\"showBackgroundColor\":false,\"value\":0,\"version\":\"R2023a\"},\"type\":\"CircularGauge\"}"  CustomBackgroundColor="{\"color\":[0.9411764705882353,0.9411764705882353,0.9411764705882353],\"show\":true}"
  Load : CustomTuningWebBlock  LabelPosition=Hide  ShowInitialText=on  Configuration="{\"components\":[{\"name\":\"LinearScaleComponent\",\"settings\":{\"bounds\":{\"max\":100,\"min\":0,\"tickInterval\":\"auto\"},\"internalTickHeightScaleFactor\":0.66,\"labelColor\":[255,255,255],\"labelFont\":{\"font\":\"Arial\",\"fontSize\":12},\"labelOffset\":0.062,\"labelTransparency\":1,\"needleImage\":{\"size\":[216,346],\"src\":\"data:image\\/jpeg;base64,\\/9j\\/60nfSlCyAAAAAAEAAEnVanVtYgAAAB5qdW1kYzJwYQARABCAAACqADibcQNjMnBhAAAANxNqdW1iAAAAR2p1bWRjMm1hABEAEIAAAKoAOJtxA3VybjpjMnBhOmZjZjA1MzM0LWQyMmQtNGI4ZS1iN2VjLWNjYWE3OTFmMGZhNgAAAAHhanVtYgAAAClqdW1kYzJhcwARABCAAACqADibcQNjMnBhLmFzc2VydGlvbnMAAAABBWp1bWIAAAApanVtZGNib3IAEQAQgAAAqgA4m3EDYzJwYS5hY3Rpb25zLnYyAAAAANRjYm9yoWdhY3Rpb25zgqNmYWN0aW9ubGMycGEuY3JlYXRlZG1zb2Z0d2FyZUFnZW50v2RuYW1lZkdQVC00b\\/ ...(+43706 chars)\",\"srcOrientation\":\"Down\"},\"needleOffset\":[0.15,-0.2634730538922156],\"needleSize\":{\"height\":0.13636363636363635,\"width\":0.2693548387096774},\"position\":[0.06363636363636363,0.2765120967741935,0.6088709677419355,0.9196022727272727],\"referencePoint\":\"auto\",\"scaleColors\":[],\"scaleColorsSize\":0.2,\"scaleDirection\":\"BT\",\"showLabels\":false,\"showMinorTicks\":0,\"showSpanLine\":false,\"showTicks\":false,\"tickColor\":[26,33,36],\"tickTransparency\":1,\"valueBarColor\":[255,255,255],\"valueBarOffset\":0.12,\"valueBarSize\":0.09,\"valueBarTransparency\":1}},{\"name\":\"BackgroundImageComponent\",\"settings\":{\"image\":{\"size\":[512,1450],\"src\":\"data:image\\/jpeg;base64,\\/9j\\/60GWSlCJAAAAAAEAAEGManVtYgAAAB5qdW1kYzJwYQARABCAAACqADibcQNjMnBhAAAANxNqdW1iAAAAR2p1bWRjMm1hABEAEIAAAKoAOJtxA3VybjpjMnBhOmZjZjA1MzM0LWQyMmQtNGI4ZS1iN2VjLWNjYWE3OTFmMGZhNgAAAAHhanVtYgAAAClqdW1kYzJhcwARABCAAACqADibcQNjMnBhLmFzc2VydGlvbnMAAAABBWp1bWIAAAApanVtZGNib3IAEQAQgAAAqgA4m3EDYzJwYS5hY3Rpb25zLnYyAAAAANRjYm9yoWdhY3Rpb25zgqNmYWN0aW9ubGMycGEuY3JlYXRlZG1zb2Z0d2FyZUFnZW50v2RuYW1lZkdQVC00b\\/ ...(+77138 chars)\",\"srcOrientation\":\"Down\"},\"position\":[0,0,1,1],\"scaleMode\":\"0\"}},{\"name\":\"ForegroundImageComponent\",\"settings\":{\"image\":{\"size\":[0,0],\"src\":\"default\",\"srcOrientation\":[]},\"isForeground\":1,\"position\":[0,0,1,1],\"scaleMode\":\"0\"}}],\"settings\":{\"BindingType\":\"param\",\"aspectRatio\":3.7777777777777777,\"backgroundColor\":[0,0,0,\"1\"],\"backgroundOffset\":0.4,\"backgroundOpacity\":1,\"fixedAspectRatio\":\"on\",\"foregroundColor\":[252,252,196],\"orientation\":\"vertical\",\"showBackgroundColor\":false,\"value\":0,\"version\":\"R2023a\"},\"type\":\"LinearGauge\"}"  CustomBackgroundColor="{\"color\":[0.0196078431372549,0.5450980392156862,0.5490196078431373],\"show\":false}"
  Load1 : CustomTuningWebBlock  LabelPosition=Hide  ShowInitialText=on  Configuration="{\"components\":[{\"name\":\"LinearScaleComponent\",\"settings\":{\"bounds\":{\"max\":4,\"min\":0.1,\"tickInterval\":\"auto\"},\"internalTickHeightScaleFactor\":0.66,\"labelColor\":[255,255,255],\"labelFont\":{\"font\":\"Arial\",\"fontSize\":12},\"labelOffset\":0.062,\"labelTransparency\":1,\"needleImage\":{\"size\":[216,346],\"src\":\"data:image\\/jpeg;base64,\\/9j\\/60nfSlCyAAAAAAEAAEnVanVtYgAAAB5qdW1kYzJwYQARABCAAACqADibcQNjMnBhAAAANxNqdW1iAAAAR2p1bWRjMm1hABEAEIAAAKoAOJtxA3VybjpjMnBhOmZjZjA1MzM0LWQyMmQtNGI4ZS1iN2VjLWNjYWE3OTFmMGZhNgAAAAHhanVtYgAAAClqdW1kYzJhcwARABCAAACqADibcQNjMnBhLmFzc2VydGlvbnMAAAABBWp1bWIAAAApanVtZGNib3IAEQAQgAAAqgA4m3EDYzJwYS5hY3Rpb25zLnYyAAAAANRjYm9yoWdhY3Rpb25zgqNmYWN0aW9ubGMycGEuY3JlYXRlZG1zb2Z0d2FyZUFnZW50v2RuYW1lZkdQVC00b\\/ ...(+43706 chars)\",\"srcOrientation\":\"Down\"},\"needleOffset\":[0.15,-0.2634730538922156],\"needleSize\":{\"height\":0.13636363636363635,\"width\":0.2693548387096774},\"position\":[0.06363636363636363,0.2765120967741935,0.6088709677419355,0.9196022727272727],\"referencePoint\":\"auto\",\"scaleColors\":[],\"scaleColorsSize\":0.2,\"scaleDirection\":\"BT\",\"showLabels\":false,\"showMinorTicks\":0,\"showSpanLine\":false,\"showTicks\":false,\"tickColor\":[26,33,36],\"tickTransparency\":1,\"valueBarColor\":[255,255,255],\"valueBarOffset\":0.12,\"valueBarSize\":0.09,\"valueBarTransparency\":1}},{\"name\":\"BackgroundImageComponent\",\"settings\":{\"image\":{\"size\":[512,1450],\"src\":\"data:image\\/jpeg;base64,\\/9j\\/60GWSlCJAAAAAAEAAEGManVtYgAAAB5qdW1kYzJwYQARABCAAACqADibcQNjMnBhAAAANxNqdW1iAAAAR2p1bWRjMm1hABEAEIAAAKoAOJtxA3VybjpjMnBhOmZjZjA1MzM0LWQyMmQtNGI4ZS1iN2VjLWNjYWE3OTFmMGZhNgAAAAHhanVtYgAAAClqdW1kYzJhcwARABCAAACqADibcQNjMnBhLmFzc2VydGlvbnMAAAABBWp1bWIAAAApanVtZGNib3IAEQAQgAAAqgA4m3EDYzJwYS5hY3Rpb25zLnYyAAAAANRjYm9yoWdhY3Rpb25zgqNmYWN0aW9ubGMycGEuY3JlYXRlZG1zb2Z0d2FyZUFnZW50v2RuYW1lZkdQVC00b\\/ ...(+77138 chars)\",\"srcOrientation\":\"Down\"},\"position\":[0,0,1,1],\"scaleMode\":\"0\"}},{\"name\":\"ForegroundImageComponent\",\"settings\":{\"image\":{\"size\":[0,0],\"src\":\"default\",\"srcOrientation\":[]},\"isForeground\":1,\"position\":[0,0,1,1],\"scaleMode\":\"0\"}}],\"settings\":{\"BindingType\":\"param\",\"aspectRatio\":3.7777777777777777,\"backgroundColor\":[0,0,0,\"1\"],\"backgroundOffset\":0.4,\"backgroundOpacity\":1,\"fixedAspectRatio\":\"on\",\"foregroundColor\":[252,252,196],\"orientation\":\"vertical\",\"showBackgroundColor\":false,\"value\":0,\"version\":\"R2023a\"},\"type\":\"LinearGauge\"}"  CustomBackgroundColor="{\"color\":[0.0196078431372549,0.5450980392156862,0.5490196078431373],\"show\":false}"
  Main Power Relay : motohawk_examples_lib/Main Power Relay Blocks/Main Power Relay  on_delay_count=2  off_delay_count=5  ecup_threshold=100  group='System | Main Power Relay'
      settings: SourceProductName=Example Blocks
  MotoTune CAN Protocol Definition : MotoHawk_Protocols_lib/MotoTune Blocks/MotoTune CAN Protocol Definition  Priority=-100  nam='MotoTuneHandler'  ref_name='CAN_1'  city_id_src=Constant  city_id=hex2dec('0B')  city_id_data_store_name='CityID'  define_rxtx_id=off  txid=hex2dec('1ff0')  rxid=hex2dec('1ff0')
      settings: SourceProductName=Protocols
  Moving Average3 : dspstat3/Moving Average  Method=Sliding window  ForgettingFactorPort=off  SpecifyWindowLength=on  WindowLength=100  OverlapLength=99  AllowArbitraryInputLength=off  ForgettingFactor=0.9  SimulateUsing=Interpreted execution
  Moving Avg filter : Subsystem
  Power gauge : CustomWebBlock  LabelPosition=Hide  ShowInitialText=on  Configuration="{\"components\":[{\"name\":\"CircularScaleComponent\",\"settings\":{\"bounds\":{\"max\":15,\"min\":0,\"tickInterval\":\"auto\"},\"direction\":\"cw\",\"flipLimits\":0,\"innerRadius\":0.75,\"internalTickHeightScaleFactor\":1,\"labelColor\":[128,128,128],\"labelFont\":{\"font\":\"Arial\",\"fontSize\":12},\"labelRadius\":0.528,\"labelTransparency\":1,\"minorTickHeightScaleFactor\":0.2,\"needleImage\":{\"size\":[200,50],\"src\":\"data:image\\/svg+xml;base64,PD94bWwgdmVyc2lvbj0iMS4wIiBlbmNvZGluZz0idXRmLTgiPz4KPCEtLSBHZW5lcmF0b3I6IEFkb2JlIElsbHVzdHJhdG9yIDI0LjEuMiwgU1ZHIEV4cG9ydCBQbHVnLUluIC4gU1ZHIFZlcnNpb246IDYuMDAgQnVpbGQgMCkgIC0tPgo8c3ZnIHZlcnNpb249IjEuMSIgaWQ9IkxheWVyXzEiIHhtbG5zPSJodHRwOi8vd3d3LnczLm9yZy8yMDAwL3N2ZyIgeG1sbnM6eGxpbms9Imh0dHA6Ly93d3cudzMub3JnLzE5OTkveGxpbmsiIHg9IjBweCIgeT0iMHB4IgoJIHZpZXdCb3g9IjAgMCAyMDAgNTAiIHN0eWxlPSJlbmFibGUtYmFja2dyb3VuZDpuZXcgMCAwIDIwMCA1MDsiIHhtbDpzcGFjZT0icHJlc2VydmUiPgo8c3R5bGUgdHlwZT0idGV4dC9jc3MiPgoJLnN0MHtmaWxsOiNFQzIxMjc7fQo8L3N0eWxlPgo8cGF0aCBjbGFzcz0ic3QwIiBkPSJNMTYyLjgsMTMuN0MxNjksNC40LDE4MS43LDEuOSwxOTEsOC4xczExLjgsMTguOSw1LjYsMjguMnMtMTguOSwxMS44LTI4LjIsNS42bDAsMAoJQzE1OS4xLDM1LjYsMTU2LjYsMjMsMTYyLjgsMTMuN0wxNjIuOCwxMy43eiBNMTY1LjgsMTUuOGMtNS4xLDcuNi0zLjEsMTcuOSw0LjYsMjNjNy42LDUuMSwxNy45LDMuMSwyMy00LjYKCWM1LjEtNy42LDMuMS0xNy45LTQuNi0yM2wwLDBDMTgxLjIsNi4yLDE3MC45LDguMiwxNjUuOCwxNS44eiIvPgo8cGF0aCBjbGFzcz0ic3QwIiBkPSJNMC40LDI1Ljl2LTMuM2wxNTktMi41Yy0wLjcsMi42LTAuNyw1LjIsMCw3LjhMMC40LDI1Ljl6Ii8+CjxjaXJjbGUgY2xhc3M9InN0MCIgY3g9IjE3OS42IiBjeT0iMjQiIHI9IjAuNyIvPgo8L3N2Zz4K\"},\"needleOffset\":[0.18464878250906522,0],\"needleOrientation\":-45,\"needleRotation\":180,\"needleSize\":{\"height\":0.11741692305346914,\"width\":0.46108337545091255},\"outerRadius\":0.9,\"position\":[0.05,0.05,0.9,0.9],\"referencePoint\":\"auto\",\"scaleAngle\":270,\"scaleAngleOffset\":135,\"scaleColors\":[],\"scaleColorsSize\":0.2,\"scaleDirection\":\"CW\",\"scalePosition\":[0,0,1,1],\"showLabels\":1,\"showMinorTicks\":1,\"showSpanLine\":1,\"showTicks\":1,\"tickColor\":[38,38,38],\"tickTransparency\":1,\"valueBarColor\":[255,0,0],\"valueBarPosition\":[0,0,1,1],\"valueBarSize\":0.2,\"valueBarTransparency\":1}},{\"name\":\"BackgroundImageComponent\",\"settings\":{\"image\":{\"size\":[500,500],\"src\":\"data:image\\/svg+xml;base64,PD94bWwgdmVyc2lvbj0iMS4wIiBlbmNvZGluZz0iVVRGLTgiIHN0YW5kYWxvbmU9Im5vIj8+CjxzdmcKICAgeG1sbnM6ZGM9Imh0dHA6Ly9wdXJsLm9yZy9kYy9lbGVtZW50cy8xLjEvIgogICB4bWxuczpjYz0iaHR0cDovL2NyZWF0aXZlY29tbW9ucy5vcmcvbnMjIgogICB4bWxuczpyZGY9Imh0dHA6Ly93d3cudzMub3JnLzE5OTkvMDIvMjItcmRmLXN5bnRheC1ucyMiCiAgIHhtbG5zOnN2Zz0iaHR0cDovL3d3dy53My5vcmcvMjAwMC9zdmciCiAgIHhtbG5zPSJodHRwOi8vd3d3LnczLm9yZy8yMDAwL3N2ZyIKICAgeG1sbnM6 ...(+9964 chars)\"},\"position\":[0,0,1,1],\"scaleMode\":\"0\"}},{\"name\":\"ForegroundImageComponent\",\"settings\":{\"image\":{\"size\":[0,0],\"src\":\"default\",\"srcOrientation\":[]},\"isForeground\":1,\"position\":[0,0,1,1],\"scaleMode\":\"0\"}}],\"settings\":{\"BindingType\":\"signal\",\"aspectRatio\":1.032258064516129,\"backgroundColor\":[0,0,0,\"1\"],\"backgroundOffset\":1,\"backgroundOpacity\":1,\"direction\":\"cw\",\"fixedAspectRatio\":\"on\",\"flipLimits\":0,\"orientation\":\"horizontal\",\"showBackgroundColor\":false,\"value\":0,\"version\":\"R2023a\"},\"type\":\"CircularGauge\"}"  CustomBackgroundColor="{\"color\":[0.9411764705882353,0.9411764705882353,0.9411764705882353],\"show\":true}"
  RPM gauge : CustomWebBlock  LabelPosition=Hide  ShowInitialText=on  Configuration="{\"components\":[{\"name\":\"CircularScaleComponent\",\"settings\":{\"bounds\":{\"max\":6000,\"min\":0,\"tickInterval\":\"auto\"},\"direction\":\"cw\",\"flipLimits\":0,\"innerRadius\":0.75,\"internalTickHeightScaleFactor\":1,\"labelColor\":[128,128,128],\"labelFont\":{\"font\":\"Arial\",\"fontSize\":12},\"labelRadius\":0.528,\"labelTransparency\":1,\"minorTickHeightScaleFactor\":0.2,\"needleImage\":{\"size\":[200,50],\"src\":\"data:image\\/svg+xml;base64,PD94bWwgdmVyc2lvbj0iMS4wIiBlbmNvZGluZz0idXRmLTgiPz4KPCEtLSBHZW5lcmF0b3I6IEFkb2JlIElsbHVzdHJhdG9yIDI0LjEuMiwgU1ZHIEV4cG9ydCBQbHVnLUluIC4gU1ZHIFZlcnNpb246IDYuMDAgQnVpbGQgMCkgIC0tPgo8c3ZnIHZlcnNpb249IjEuMSIgaWQ9IkxheWVyXzEiIHhtbG5zPSJodHRwOi8vd3d3LnczLm9yZy8yMDAwL3N2ZyIgeG1sbnM6eGxpbms9Imh0dHA6Ly93d3cudzMub3JnLzE5OTkveGxpbmsiIHg9IjBweCIgeT0iMHB4IgoJIHZpZXdCb3g9IjAgMCAyMDAgNTAiIHN0eWxlPSJlbmFibGUtYmFja2dyb3VuZDpuZXcgMCAwIDIwMCA1MDsiIHhtbDpzcGFjZT0icHJlc2VydmUiPgo8c3R5bGUgdHlwZT0idGV4dC9jc3MiPgoJLnN0MHtmaWxsOiNFQzIxMjc7fQo8L3N0eWxlPgo8cGF0aCBjbGFzcz0ic3QwIiBkPSJNMTYyLjgsMTMuN0MxNjksNC40LDE4MS43LDEuOSwxOTEsOC4xczExLjgsMTguOSw1LjYsMjguMnMtMTguOSwxMS44LTI4LjIsNS42bDAsMAoJQzE1OS4xLDM1LjYsMTU2LjYsMjMsMTYyLjgsMTMuN0wxNjIuOCwxMy43eiBNMTY1LjgsMTUuOGMtNS4xLDcuNi0zLjEsMTcuOSw0LjYsMjNjNy42LDUuMSwxNy45LDMuMSwyMy00LjYKCWM1LjEtNy42LDMuMS0xNy45LTQuNi0yM2wwLDBDMTgxLjIsNi4yLDE3MC45LDguMiwxNjUuOCwxNS44eiIvPgo8cGF0aCBjbGFzcz0ic3QwIiBkPSJNMC40LDI1Ljl2LTMuM2wxNTktMi41Yy0wLjcsMi42LTAuNyw1LjIsMCw3LjhMMC40LDI1Ljl6Ii8+CjxjaXJjbGUgY2xhc3M9InN0MCIgY3g9IjE3OS42IiBjeT0iMjQiIHI9IjAuNyIvPgo8L3N2Zz4K\"},\"needleOffset\":[0.18464878250906522,0],\"needleOrientation\":-45,\"needleRotation\":180,\"needleSize\":{\"height\":0.11741692305346914,\"width\":0.46108337545091255},\"outerRadius\":0.9,\"position\":[0.05,0.05,0.9,0.9],\"referencePoint\":\"auto\",\"scaleAngle\":270,\"scaleAngleOffset\":135,\"scaleColors\":[],\"scaleColorsSize\":0.2,\"scaleDirection\":\"CW\",\"scalePosition\":[0,0,1,1],\"showLabels\":1,\"showMinorTicks\":1,\"showSpanLine\":1,\"showTicks\":1,\"tickColor\":[38,38,38],\"tickTransparency\":1,\"valueBarColor\":[255,0,0],\"valueBarPosition\":[0,0,1,1],\"valueBarSize\":0.2,\"valueBarTransparency\":1}},{\"name\":\"BackgroundImageComponent\",\"settings\":{\"image\":{\"size\":[500,500],\"src\":\"data:image\\/svg+xml;base64,PD94bWwgdmVyc2lvbj0iMS4wIiBlbmNvZGluZz0iVVRGLTgiIHN0YW5kYWxvbmU9Im5vIj8+CjxzdmcKICAgeG1sbnM6ZGM9Imh0dHA6Ly9wdXJsLm9yZy9kYy9lbGVtZW50cy8xLjEvIgogICB4bWxuczpjYz0iaHR0cDovL2NyZWF0aXZlY29tbW9ucy5vcmcvbnMjIgogICB4bWxuczpyZGY9Imh0dHA6Ly93d3cudzMub3JnLzE5OTkvMDIvMjItcmRmLXN5bnRheC1ucyMiCiAgIHhtbG5zOnN2Zz0iaHR0cDovL3d3dy53My5vcmcvMjAwMC9zdmciCiAgIHhtbG5zPSJodHRwOi8vd3d3LnczLm9yZy8yMDAwL3N2ZyIKICAgeG1sbnM6 ...(+9964 chars)\"},\"position\":[0,0,1,1],\"scaleMode\":\"0\"}},{\"name\":\"ForegroundImageComponent\",\"settings\":{\"image\":{\"size\":[0,0],\"src\":\"default\",\"srcOrientation\":[]},\"isForeground\":1,\"position\":[0,0,1,1],\"scaleMode\":\"0\"}}],\"settings\":{\"BindingType\":\"signal\",\"aspectRatio\":1.032258064516129,\"backgroundColor\":[0,0,0,\"1\"],\"backgroundOffset\":1,\"backgroundOpacity\":1,\"direction\":\"cw\",\"fixedAspectRatio\":\"on\",\"flipLimits\":0,\"orientation\":\"horizontal\",\"showBackgroundColor\":false,\"value\":0,\"version\":\"R2023a\"},\"type\":\"CircularGauge\"}"  CustomBackgroundColor="{\"color\":[0.9411764705882353,0.9411764705882353,0.9411764705882353],\"show\":true}"
  Rate Transition : RateTransition
  Subsystem : Subsystem
  Subsystem1 : Subsystem
  Torque : CustomWebBlock  LabelPosition=Hide  ShowInitialText=on  Configuration="{\"components\":[{\"name\":\"CircularScaleComponent\",\"settings\":{\"bounds\":{\"max\":40,\"min\":0,\"tickInterval\":\"auto\"},\"direction\":\"cw\",\"flipLimits\":0,\"innerRadius\":0.75,\"internalTickHeightScaleFactor\":1,\"labelColor\":[128,128,128],\"labelFont\":{\"font\":\"Arial\",\"fontSize\":12},\"labelRadius\":0.528,\"labelTransparency\":1,\"minorTickHeightScaleFactor\":0.2,\"needleImage\":{\"size\":[200,50],\"src\":\"data:image\\/svg+xml;base64,PD94bWwgdmVyc2lvbj0iMS4wIiBlbmNvZGluZz0idXRmLTgiPz4KPCEtLSBHZW5lcmF0b3I6IEFkb2JlIElsbHVzdHJhdG9yIDI0LjEuMiwgU1ZHIEV4cG9ydCBQbHVnLUluIC4gU1ZHIFZlcnNpb246IDYuMDAgQnVpbGQgMCkgIC0tPgo8c3ZnIHZlcnNpb249IjEuMSIgaWQ9IkxheWVyXzEiIHhtbG5zPSJodHRwOi8vd3d3LnczLm9yZy8yMDAwL3N2ZyIgeG1sbnM6eGxpbms9Imh0dHA6Ly93d3cudzMub3JnLzE5OTkveGxpbmsiIHg9IjBweCIgeT0iMHB4IgoJIHZpZXdCb3g9IjAgMCAyMDAgNTAiIHN0eWxlPSJlbmFibGUtYmFja2dyb3VuZDpuZXcgMCAwIDIwMCA1MDsiIHhtbDpzcGFjZT0icHJlc2VydmUiPgo8c3R5bGUgdHlwZT0idGV4dC9jc3MiPgoJLnN0MHtmaWxsOiNFQzIxMjc7fQo8L3N0eWxlPgo8cGF0aCBjbGFzcz0ic3QwIiBkPSJNMTYyLjgsMTMuN0MxNjksNC40LDE4MS43LDEuOSwxOTEsOC4xczExLjgsMTguOSw1LjYsMjguMnMtMTguOSwxMS44LTI4LjIsNS42bDAsMAoJQzE1OS4xLDM1LjYsMTU2LjYsMjMsMTYyLjgsMTMuN0wxNjIuOCwxMy43eiBNMTY1LjgsMTUuOGMtNS4xLDcuNi0zLjEsMTcuOSw0LjYsMjNjNy42LDUuMSwxNy45LDMuMSwyMy00LjYKCWM1LjEtNy42LDMuMS0xNy45LTQuNi0yM2wwLDBDMTgxLjIsNi4yLDE3MC45LDguMiwxNjUuOCwxNS44eiIvPgo8cGF0aCBjbGFzcz0ic3QwIiBkPSJNMC40LDI1Ljl2LTMuM2wxNTktMi41Yy0wLjcsMi42LTAuNyw1LjIsMCw3LjhMMC40LDI1Ljl6Ii8+CjxjaXJjbGUgY2xhc3M9InN0MCIgY3g9IjE3OS42IiBjeT0iMjQiIHI9IjAuNyIvPgo8L3N2Zz4K\"},\"needleOffset\":[0.18464878250906522,0],\"needleOrientation\":-45,\"needleRotation\":180,\"needleSize\":{\"height\":0.11741692305346914,\"width\":0.46108337545091255},\"outerRadius\":0.9,\"position\":[0.05,0.05,0.9,0.9],\"referencePoint\":\"auto\",\"scaleAngle\":270,\"scaleAngleOffset\":135,\"scaleColors\":[],\"scaleColorsSize\":0.2,\"scaleDirection\":\"CW\",\"scalePosition\":[0,0,1,1],\"showLabels\":1,\"showMinorTicks\":1,\"showSpanLine\":1,\"showTicks\":1,\"tickColor\":[38,38,38],\"tickTransparency\":1,\"valueBarColor\":[255,0,0],\"valueBarPosition\":[0,0,1,1],\"valueBarSize\":0.2,\"valueBarTransparency\":1}},{\"name\":\"BackgroundImageComponent\",\"settings\":{\"image\":{\"size\":[500,500],\"src\":\"data:image\\/svg+xml;base64,PD94bWwgdmVyc2lvbj0iMS4wIiBlbmNvZGluZz0iVVRGLTgiIHN0YW5kYWxvbmU9Im5vIj8+CjxzdmcKICAgeG1sbnM6ZGM9Imh0dHA6Ly9wdXJsLm9yZy9kYy9lbGVtZW50cy8xLjEvIgogICB4bWxuczpjYz0iaHR0cDovL2NyZWF0aXZlY29tbW9ucy5vcmcvbnMjIgogICB4bWxuczpyZGY9Imh0dHA6Ly93d3cudzMub3JnLzE5OTkvMDIvMjItcmRmLXN5bnRheC1ucyMiCiAgIHhtbG5zOnN2Zz0iaHR0cDovL3d3dy53My5vcmcvMjAwMC9zdmciCiAgIHhtbG5zPSJodHRwOi8vd3d3LnczLm9yZy8yMDAwL3N2ZyIKICAgeG1sbnM6 ...(+9964 chars)\"},\"position\":[0,0,1,1],\"scaleMode\":\"0\"}},{\"name\":\"ForegroundImageComponent\",\"settings\":{\"image\":{\"size\":[0,0],\"src\":\"default\",\"srcOrientation\":[]},\"isForeground\":1,\"position\":[0,0,1,1],\"scaleMode\":\"0\"}}],\"settings\":{\"BindingType\":\"signal\",\"aspectRatio\":1.032258064516129,\"backgroundColor\":[0,0,0,\"1\"],\"backgroundOffset\":1,\"backgroundOpacity\":1,\"direction\":\"cw\",\"fixedAspectRatio\":\"on\",\"flipLimits\":0,\"orientation\":\"horizontal\",\"showBackgroundColor\":false,\"value\":0,\"version\":\"R2023a\"},\"type\":\"CircularGauge\"}"  CustomBackgroundColor="{\"color\":[0.9411764705882353,0.9411764705882353,0.9411764705882353],\"show\":true}"
  h2 request : Constant  Value=0
  motohawk_TitleBlock : motohawk_annotations_lib/motohawk_TitleBlock  BlockType_='Mototron_Title_Block'  ttl="[        strrep(get_param(bdroot, 'Description') , '_', '\\_')  '\\newline\\rm'        'Top-level root of model:  '   strrep(bdroot, '_', '\\_') '.mdl'        ]"  copyright="'THE INFORMATION CONTAINED IN THIS\\newlineDRAWING IS THE SOLE PROPERTY OF\\newlineWOODWARD.  ANY REPRODUCTION IN\\newline PART OR AS A WHOLE WITHOUT THE\\newlineWRITTEN PERMISSION OF WOODWARD\\newline IS PROHIBITED.\\fontsize{16}\\rm\\copyright\\rm\\fontsize{10} 2017'"  address='\fontsize{22}\it\fontname{Arial Black}Woodward \fontname{Arial}\fontsize{10}\newline1081 Woodward Way, Fort Collins, CO, 80524\newlinemcs.woodward.com'  image_file='mh.jpg'  pretty_print=on  edit_text="[strrep(get_param(bdroot, 'Description') , '_', '\\_')  '\\newline\\rm''Top-level root of model:  '   strrep(bdroot, '_', '\\_') '.mdl']"  edit_as=5
      settings: SourceProductName=MotoHawk Annotations
  motohawk_app_monitor : MotoHawk_lib/System Debug Blocks/motohawk_app_monitor  fgnd_stack_margin=512  fgnd_angle_stack_margin=256  bgnd_stack_margin=256  idle_stack_margin=256  irq_stack_margin=128  heap_margin=256  cpu_margin=10  init_enable=Enabled  pause_point=Do Not Pause on Startup
      settings: SourceProductName=MotoHawk
  motohawk_code_coverage_mgr : MotoHawk_lib/Extra Development Blocks/motohawk_code_coverage_mgr  codegen=Always Generate Code Coverage Code  group='System | Code Coverage'
      settings: SourceProductName=MotoHawk
  motohawk_target_def1 : MotoHawk_lib/motohawk_target_def  Priority=-65535  target=ECU555-48-0403  layout=DEV  fptype=single (32 bits)  use_target_os_config=off  target_os=ControlCore  default_target_os=Classic ControlCore  fgnd_stack_size=4*1024  fgnd_angle_stack_size=4*1024  bgnd_stack_size=4*1024  idle_stack_size=4*1024  irq_stack_size=4*1024  app_int_stack_size=1024  shutdown_stack_size=1024  heap_size=4*1024  show_margins=off  fgnd_stack_margin=(3*1024) * 0.1  fgnd_angle_stack_margin=0  bgnd_stack_margin=(2*1024) * 0.1  idle_stack_margin=(1024) * 0.1  irq_stack_margin=(1536) * 0.1  app_int_stack_margin=(1024) * 0.1  shutdown_stack_margin=(1024) * 0.1  heap_margin=(4*1024) * 0.1  comp_name=bdroot  comp_img='KVASER_CAN_USB.jpg'  comp_security=No Encryption  comp_build_pass='mhbuild'  comp_sim_pass='mhsim'  comp_multi=off  show_filenames=off  dll_name=motohawk_trunc_name(bdroot, ['_' motohawk_build_version], 50)  srz_name=motohawk_trunc_name(bdroot, ['_' motohawk_build_version], 50)  build_dir='.'  comp_dir='.'
      settings: SourceProductName=MotoHawk
  motohawk_trigger : MotoHawk_lib/Trigger Blocks/motohawk_trigger  Tag=Trigger  Priority=0  trig_name=[]  trigger=FGND_RTI_PERIODIC  priority_order=0  inherited=off  run_disabled=off  override_app_monitor=off  target=ECU555_48_0403
      settings: SourceProductName=MotoHawk
  motohawk_trigger1 : MotoHawk_lib/Trigger Blocks/motohawk_trigger  Tag=Trigger  Priority=0  trig_name=[]  trigger=BGND_BASE_PERIODIC  priority_order=0  inherited=off  run_disabled=off  override_app_monitor=off  target=ECU555_48_0403
      settings: SourceProductName=MotoHawk
  motohawk_trigger_def : MotoHawk_lib/Trigger Blocks/motohawk_trigger_def  fgnd_rti_rate=5000  suppress_fgnd_rti_warning=off  bgnd_base_multiple=20  read_level=1  write_level=1  mototune_group='System | System Config | Trigger Config'
      settings: SourceProductName=MotoHawk
  AFR & IMEP : Scope
  BSFC : Scope
  Energy : Scope
  Power & Torque : Scope
  RPM : Scope
  Scope{,1..5} (6 alike) : Scope
  Temps : Scope
  wires:
  motohawk_trigger/1 -> Foreground/Trigger
  Foreground/1(Out1) -> Bus Selector/1
  Subsystem/1(Out1) -> Foreground/1(FMU), Rate Transition/1
  h2 request/1 -> Subsystem/11(In8)
  Bus Selector/1 -> FMU/1  "<InjM_D>"
  FMU/8 -> Subsystem/8(MF_IA)
  FMU/9 -> Moving Average3/1  "IAT"
  FMU/10 -> Subsystem/10(MAP)  "MAP"
  FMU/1 -> Moving Avg filter/1(AFR)  "AFR"
  FMU/2 -> Moving Avg filter/2(IMEP)  "IMEP"
  FMU/3 -> Moving Avg filter/3(EGT)  "EGT"
  FMU/4 -> Moving Avg filter/4(BSFC)  "BSFC"
  FMU/5 -> Moving Avg filter/5(Torque)  "Torque"
  FMU/6 -> Moving Avg filter/6(PWR)  "PWR"
  FMU/7 -> Moving Avg filter/7(RPM)  "RPM"
  Moving Avg filter/1(Out1) -> Subsystem/1(AFR)  "AFR"
  Moving Avg filter/2(Out2) -> Subsystem/2(IMEP)  "IMEP"
  Moving Avg filter/3(Out3) -> Subsystem/3(EGT)  "EGT"
  Moving Avg filter/4(Out4) -> Subsystem/4(BSFC)  "BSFC"
  Moving Avg filter/5(Out5) -> Subsystem/5(Torque)  "Torque"
  Moving Avg filter/6(Out6) -> Subsystem/6(PWR)  "PWR"
  Moving Avg filter/7(Out7) -> Subsystem/7(RPM)  "RPM"
  motohawk_trigger1/1 -> Background/Trigger
  Rate Transition/1 -> Background/1(FMU)
  Moving Average3/1 -> Subsystem/9(IAT)  "IAT"
  FMU/11 -> Subsystem1/1(In1)
  Bus Selector/2 -> FMU/2  "<inj_H2>"
  FMU/12 -> Subsystem1/2(In3)
  Constant2/1 -> FMU/3
